simulink model "cordic"  (R2024b)
settings: Solver=VariableStepAuto  StartTime=0.0  StopTime=4e-6  RelTol=1e-3
libraries: fillib x1
settings Model: Creator=ETLCLab-Tesisti  LastModifiedBy=ETLCLab-Tesisti

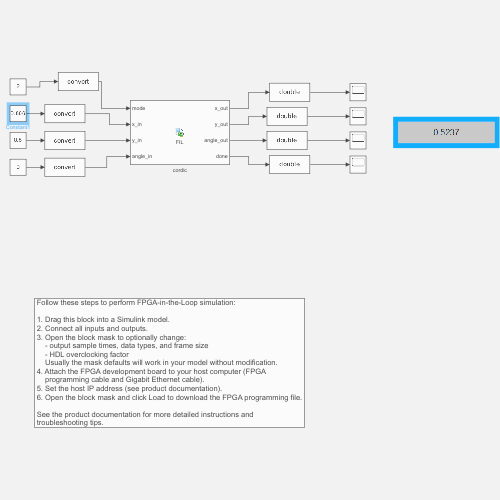
[thumbnail: Simulink's stored preview of the top-level diagram]
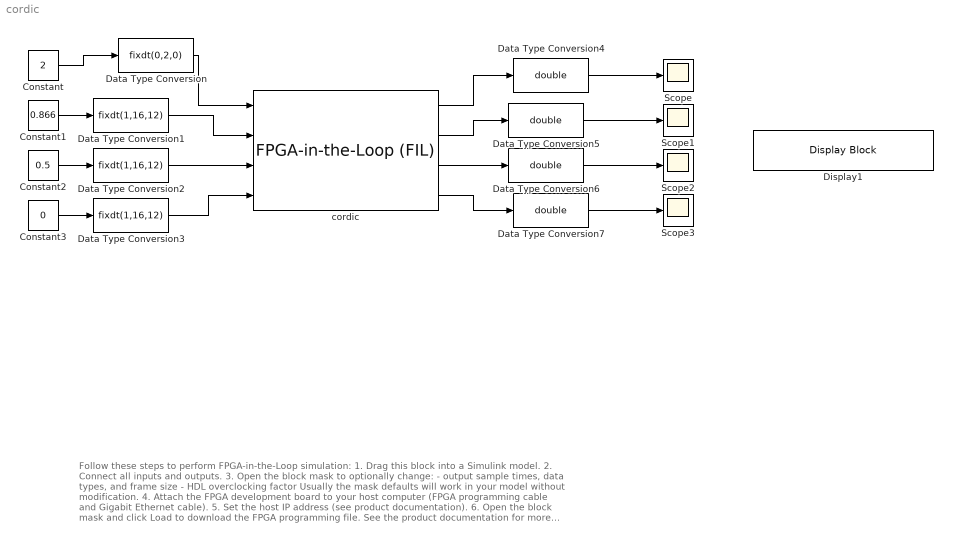
== system cordic ==
  note: Follow these steps to perform FPGA-in-the-Loop simulation:
      |
      | 1. Drag this block into a Simulink model.
      | 2. Connect all inputs and outputs.
      | 3. Open the block mask to optionally change:
      |     - output sample times, data types, and frame size
      |     - HDL overclocking factor
      |     Usually the mask defaults will work in your model without modification.
      | 4. Attach the FPGA development board to your host computer (FPGA
      |     programming cable and Gigabit Ethernet cable).
      | 5. Set the host IP address (see product documentation).
      | 6. Open the block mask and click Load to download the FPGA programming file.
      |
      | See the product documentation for more detailed instructions and
      | troubleshooting tips.
  Constant : Constant  Value=2  OutDataTypeStr=double  SampleTime=1/25e6
  Constant1 : Constant  Value=0.866  SampleTime=1/25e6
  Constant2 : Constant  Value=0.5  SampleTime=1/25e6
  Constant3 : Constant  Value=0  SampleTime=1/25e6
  Data Type Conversion : DataTypeConversion  OutDataTypeStr=fixdt(0,2,0)  RndMeth=Floor
  Data Type Conversion1 : DataTypeConversion  OutDataTypeStr=fixdt(1,16,12)  RndMeth=Floor
  Data Type Conversion2 : DataTypeConversion  OutDataTypeStr=fixdt(1,16,12)  RndMeth=Floor
  Data Type Conversion3 : DataTypeConversion  OutDataTypeStr=fixdt(1,16,12)  RndMeth=Floor
  Data Type Conversion{4..7} (4 alike) : DataTypeConversion  OutDataTypeStr=double  RndMeth=Floor
  Display1 : DisplayBlock  LabelPosition=Hide  Transparency=1
  Scope{,1..3} (4 alike) : Scope
  cordic : fillib/FPGA-in-the-Loop (FIL)  ForceInterfaceUpdate=0.09754
  wires:
  Data Type Conversion1/1 -> cordic/2
  Data Type Conversion3/1 -> cordic/4
  Data Type Conversion/1 -> cordic/1
  Constant1/1 -> Data Type Conversion1/1
  Data Type Conversion2/1 -> cordic/3
  Constant3/1 -> Data Type Conversion3/1
  Constant2/1 -> Data Type Conversion2/1
  Constant/1 -> Data Type Conversion/1
  Data Type Conversion5/1 -> Scope1/1
  cordic/3 -> Data Type Conversion6/1
  Data Type Conversion7/1 -> Scope3/1
  cordic/4 -> Data Type Conversion7/1
  Data Type Conversion4/1 -> Scope/1
  Data Type Conversion6/1 -> Scope2/1
  cordic/1 -> Data Type Conversion4/1
  cordic/2 -> Data Type Conversion5/1
